simulink model "control_attempt_dofmodel"  (R2020b)
settings: Solver=VariableStepAuto  StartTime=0.0  StopTime=120  FixedStep=0.0001
values from neighbouring files (symbols this model uses):
  g = -9.81    [Variables.m]
undefined symbols (not defined in the file or in its folder): b, ct, Jm, Ke, Kt, L, m, Rm
libraries: pid_lib x2, shared6dof x1
settings Model: Creator=Josh_  LastModifiedBy=maria
settings SolverCC: MaxConsecutiveMinStep=5
settings DataIOCC: SaveFormat=Array  ReturnWorkspaceOutputs=off

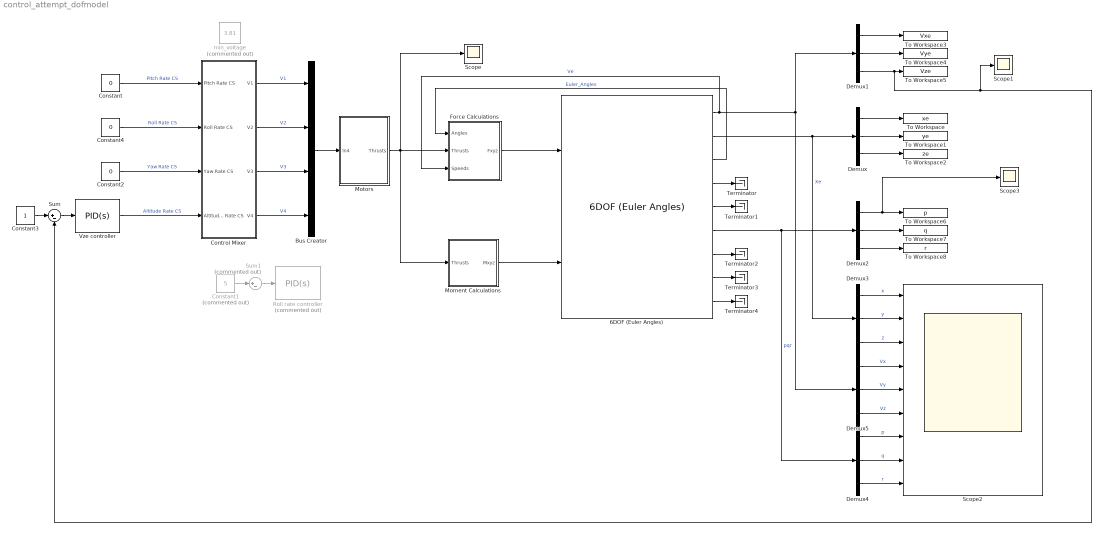
== system control_attempt_dofmodel ==
  6DOF (Euler Angles) : shared6dof/6DOF (Euler Angles)  units=Metric (MKS)  mtype=Fixed  rep=Euler Angles  xme_0=[0 0 0]  Vm_0=[0 0 0]  eul_0=[0 0 0]  pm_0=[0 0 0]  mass_0=m  mass_e=0.5  mass_f=2.0  inertia=eye(3)  inertia_e=eye(3)  inertia_f=2*eye(3)  k_quat=1.0  vre_flag=on  abi_flag=on  aMode=0  xme_statename=''  Vm_statename=''  eul_statename=''  quat_statename=''  pm_statename=''  mass_statename=''
      settings: SourceProductBaseCode=AE,PW,MT,UV,VE,VP
  Bus Creator : BusCreator  Inputs=4
  Constant : Constant  Value=0
  Constant1 : Constant  Commented=on  Value=5
  Constant2 : Constant  Value=0
  Constant3 : Constant
  Constant4 : Constant  Value=0
  Control Mixer : Subsystem
  Demux{,1..5} (6 alike) : Demux  Outputs=3
  Force Calculations : Subsystem
  Moment Calculations : Subsystem
  Motors : Subsystem
  Roll rate controller : pid_lib/PID Controller  Commented=on  Controller=PID  Form=Parallel  TimeDomain=Continuous-time  UseExternalTs=off  SampleTime=-1  IntegratorMethod=Forward Euler  FilterMethod=Forward Euler  ControllerParametersSource=internal  P=249903802210.165  I=8046092299.48993  D=1724573422053.39  UseFilter=on  N=630.713138898879  TunerSelectOption=Transfer Function Based (PID Tuner App)  InitialConditionSource=internal  InitialConditionForIntegrator=0  InitialConditionForFilter=0  DifferentiatorICPrevScaledInput=0  ExternalReset=none  TrackingMode=off  Kt=1  LimitOutput=off  SatLimitsSource=internal  UpperSaturationLimit=inf  LowerSaturationLimit=-inf  LinearizeAsGain=on  AntiWindupMode=none  Kb=1  POutMin=[]  POutMax=[]  IOutMin=[]  IOutMax=[]  DOutMin=[]  DOutMax=[]  NOutMin=[]  NOutMax=[]  SumOutMin=[]  SumOutMax=[]  SaturationOutMin=[]  SaturationOutMax=[]  PParamMin=[]  PParamMax=[]  IParamMin=[]  IParamMax=[]  DParamMin=[]  DParamMax=[]  NParamMin=[]  NParamMax=[]  KbParamMin=[]  KbParamMax=[]  KtParamMin=[]  KtParamMax=[]  KbOutMin=[]  KbOutMax=[]  KtOutMin=[]  KtOutMax=[]  IntegratorOutMin=[]  IntegratorOutMax=[]  FilterOutMin=[]  FilterOutMax=[]  SumI1OutMin=[]  SumI1OutMax=[]  SumI2OutMin=[]  SumI2OutMax=[]  SumI3OutMin=[]  SumI3OutMax=[]  SumI4OutMin=[]  SumI4OutMax=[]  SumDOutMin=[]  SumDOutMax=[]  DifferentiatorOutMin=[]  DifferentiatorOutMax=[]  FilterDiffOutCoefMin=[]  FilterDiffOutCoefMax=[]  ReciprocalOutMin=[]  ReciprocalOutMax=[]  SumDenOutMin=[]  SumDenOutMax=[]  SumNumOutMin=[]  SumNumOutMax=[]  DivideOutMin=[]  DivideOutMax=[]  UdiffTsProdOutMin=[]  UdiffTsProdOutMax=[]  NTsProdOutMin=[]  NTsProdOutMax=[]  UintegralTsProdOutMin=[]  UintegralTsProdOutMax=[]  UngainTsProdOutMin=[]  UngainTsProdOutMax=[]  IntegratorContinuousStateAttributes=''  IntegratorStateMustResolveToSignalObject=off  IntegratorRTWStateStorageClass=Auto  FilterContinuousStateAttributes=''  FilterStateMustResolveToSignalObject=off  FilterRTWStateStorageClass=Auto  ParallelPVariant=InternalParameters  IdealPVariant=Disabled  IVariant=InternalParameters  DVariant=InternalParameters  IntegratorVariant=Continuous  SatVariant=Disabled  AWVariant=Passthrough  PCopyVariant=Disabled  TRVariant=Disabled  FdbkBlocksVariant=Forward  IdealPFdbkVariant=Disabled  SatFdbkVariant=Disabled  DerivativeFilterVariant=ContFilter  NVariant=InternalParameters  NCopyVariant=Disabled  FilterICVariant=InternalICsFilter  IntegratorICVariant=InternalICs  ExternalResetVariant=Disabled  TRSumVariant=Passthrough  SumFdbkVariant=Disabled  SumVariant=Sum_PID  TsampFilterVariant=InternalTs  TsampNgainVariant=Passthrough  TsampIntegralVariant=Passthrough  ExternalSaturationOutDataTypeStr=Inherit: Same as second input
  Scope : Scope
  Scope1 : Scope
  Scope2 : Scope  NumInputPorts=9
  Scope3 : Scope
  Sum : Sum  Inputs=|+-
  Sum1 : Sum  Commented=on  Inputs=|+-
  Terminator{,1..4} (5 alike) : Terminator
  To Workspace : ToWorkspace  VariableName=xe  SampleTime=-1
  To Workspace1 : ToWorkspace  VariableName=ye  SampleTime=-1
  To Workspace2 : ToWorkspace  VariableName=ze  SampleTime=-1
  To Workspace3 : ToWorkspace  VariableName=Vxe  SampleTime=-1
  To Workspace4 : ToWorkspace  VariableName=Vye  SampleTime=-1
  To Workspace5 : ToWorkspace  VariableName=Vze  SampleTime=-1
  To Workspace6 : ToWorkspace  VariableName=p  SampleTime=-1
  To Workspace7 : ToWorkspace  VariableName=q  SampleTime=-1
  To Workspace8 : ToWorkspace  VariableName=r  SampleTime=-1
  Vze controller : pid_lib/PID Controller  Controller=PID  Form=Parallel  TimeDomain=Continuous-time  UseExternalTs=off  SampleTime=-1  IntegratorMethod=Forward Euler  FilterMethod=Forward Euler  ControllerParametersSource=internal  P=0.555  I=0.018  D=3.728  UseFilter=on  N=647.736587390862  TunerSelectOption=Transfer Function Based (PID Tuner App)  InitialConditionSource=internal  InitialConditionForIntegrator=0  InitialConditionForFilter=0  DifferentiatorICPrevScaledInput=0  ExternalReset=none  TrackingMode=off  Kt=1  LimitOutput=off  SatLimitsSource=internal  UpperSaturationLimit=inf  LowerSaturationLimit=-inf  LinearizeAsGain=on  AntiWindupMode=none  Kb=1  POutMin=[]  POutMax=[]  IOutMin=[]  IOutMax=[]  DOutMin=[]  DOutMax=[]  NOutMin=[]  NOutMax=[]  SumOutMin=[]  SumOutMax=[]  SaturationOutMin=[]  SaturationOutMax=[]  PParamMin=[]  PParamMax=[]  IParamMin=[]  IParamMax=[]  DParamMin=[]  DParamMax=[]  NParamMin=[]  NParamMax=[]  KbParamMin=[]  KbParamMax=[]  KtParamMin=[]  KtParamMax=[]  KbOutMin=[]  KbOutMax=[]  KtOutMin=[]  KtOutMax=[]  IntegratorOutMin=[]  IntegratorOutMax=[]  FilterOutMin=[]  FilterOutMax=[]  SumI1OutMin=[]  SumI1OutMax=[]  SumI2OutMin=[]  SumI2OutMax=[]  SumI3OutMin=[]  SumI3OutMax=[]  SumI4OutMin=[]  SumI4OutMax=[]  SumDOutMin=[]  SumDOutMax=[]  DifferentiatorOutMin=[]  DifferentiatorOutMax=[]  FilterDiffOutCoefMin=[]  FilterDiffOutCoefMax=[]  ReciprocalOutMin=[]  ReciprocalOutMax=[]  SumDenOutMin=[]  SumDenOutMax=[]  SumNumOutMin=[]  SumNumOutMax=[]  DivideOutMin=[]  DivideOutMax=[]  UdiffTsProdOutMin=[]  UdiffTsProdOutMax=[]  NTsProdOutMin=[]  NTsProdOutMax=[]  UintegralTsProdOutMin=[]  UintegralTsProdOutMax=[]  UngainTsProdOutMin=[]  UngainTsProdOutMax=[]  IntegratorContinuousStateAttributes=''  IntegratorStateMustResolveToSignalObject=off  IntegratorRTWStateStorageClass=Auto  FilterContinuousStateAttributes=''  FilterStateMustResolveToSignalObject=off  FilterRTWStateStorageClass=Auto  ParallelPVariant=InternalParameters  IdealPVariant=Disabled  IVariant=InternalParameters  DVariant=InternalParameters  IntegratorVariant=Continuous  SatVariant=Disabled  AWVariant=Passthrough  PCopyVariant=Disabled  TRVariant=Disabled  FdbkBlocksVariant=Forward  IdealPFdbkVariant=Disabled  SatFdbkVariant=Disabled  DerivativeFilterVariant=ContFilter  NVariant=InternalParameters  NCopyVariant=Disabled  FilterICVariant=InternalICsFilter  IntegratorICVariant=InternalICs  ExternalResetVariant=Disabled  TRSumVariant=Passthrough  SumFdbkVariant=Disabled  SumVariant=Sum_PID  TsampFilterVariant=InternalTs  TsampNgainVariant=Passthrough  TsampIntegralVariant=Passthrough  ExternalSaturationOutDataTypeStr=Inherit: Same as second input
  min_voltage : Constant  Commented=on  Value=3.81
  wires:
  Demux4/1 -> Scope2/7  "p"
  Demux3/3 -> Scope2/3  "z"
  Demux4/2 -> Scope2/8  "q"
  Demux4/3 -> Scope2/9  "r"
  Demux5/2 -> Scope2/5  "Vy"
  Demux2/1 -> Scope3/1, To Workspace6/1
  Demux3/2 -> Scope2/2  "y"
  Constant/1 -> Control Mixer/1(Pitch Rate CS)  "Pitch Rate CS"
  Vze controller/1 -> Control Mixer/4(Altitude Rate CS)  "Altitude Rate CS"
  Demux3/1 -> Scope2/1  "x"
  6DOF (Euler Angles)/6 -> Demux4/1, Demux2/1  "pqr"
  Demux5/1 -> Scope2/4  "Vx"
  Demux2/3 -> To Workspace8/1
  Demux2/2 -> To Workspace7/1
  Control Mixer/4(V4) -> Bus Creator/4  "V4"
  Demux5/3 -> Scope2/6  "Vz"
  Control Mixer/3(V3) -> Bus Creator/3  "V3"
  Demux/1 -> To Workspace/1
  Constant2/1 -> Control Mixer/3(Yaw Rate CS)  "Yaw Rate CS"
  Demux1/2 -> To Workspace4/1
  Demux1/1 -> To Workspace3/1
  Motors/1(Thrusts) -> Moment Calculations/1(Thrusts), Force Calculations/2(Thrusts), Scope/1
  Control Mixer/1(V1) -> Bus Creator/1  "V1"
  Demux1/3 -> Scope1/1, Sum/2, To Workspace5/1
  Control Mixer/2(V2) -> Bus Creator/2  "V2"
  Bus Creator/1 -> Motors/1(In4)
  Demux/3 -> To Workspace2/1
  Force Calculations/1(Fxyz) -> 6DOF (Euler Angles)/1
  Demux/2 -> To Workspace1/1
  6DOF (Euler Angles)/2 -> Demux3/1, Demux/1  "Xe"
  Moment Calculations/1(Mxyz) -> 6DOF (Euler Angles)/2
  6DOF (Euler Angles)/3 -> Force Calculations/1(Angles)  "Euler_Angles"
  6DOF (Euler Angles)/1 -> Force Calculations/3(Speeds), Demux5/1, Demux1/1  "Ve"
  Constant3/1 -> Sum/1
  Sum/1 -> Vze controller/1
  6DOF (Euler Angles)/4 -> Terminator/1
  6DOF (Euler Angles)/5 -> Terminator1/1
  6DOF (Euler Angles)/7 -> Terminator2/1
  6DOF (Euler Angles)/8 -> Terminator3/1
  6DOF (Euler Angles)/9 -> Terminator4/1
  Sum1/1 -> Roll rate controller/1
  Constant1/1 -> Sum1/1
  Constant4/1 -> Control Mixer/2(Roll Rate CS)  "Roll Rate CS"

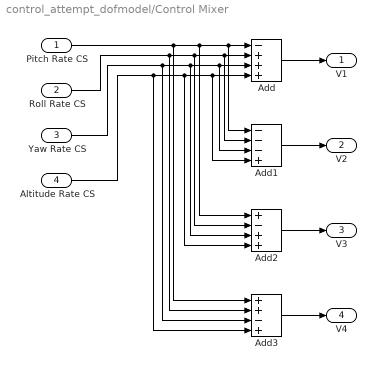
== system control_attempt_dofmodel/Control Mixer ==
  Pitch Rate CS : Inport
  Roll Rate CS : Inport  Port=2
  Yaw Rate CS : Inport  Port=3
  Altitude Rate CS : Inport  Port=4
  Add : Sum  Inputs=-+++
  Add1 : Sum  Inputs=---+
  Add2 : Sum  Inputs=+-++
  Add3 : Sum  Inputs=++-+
  V1 : Outport
  V2 : Outport  Port=2
  V3 : Outport  Port=3
  V4 : Outport  Port=4
  wires:
  Pitch Rate CS/1 -> Add1/1, Add/1, Add2/1, Add3/1
  Roll Rate CS/1 -> Add1/2, Add/2, Add2/2, Add3/2
  Yaw Rate CS/1 -> Add3/3, Add1/3, Add/3, Add2/3
  Altitude Rate CS/1 -> Add2/4, Add1/4, Add/4, Add3/4
  Add/1 -> V1/1
  Add1/1 -> V2/1
  Add2/1 -> V3/1
  Add3/1 -> V4/1

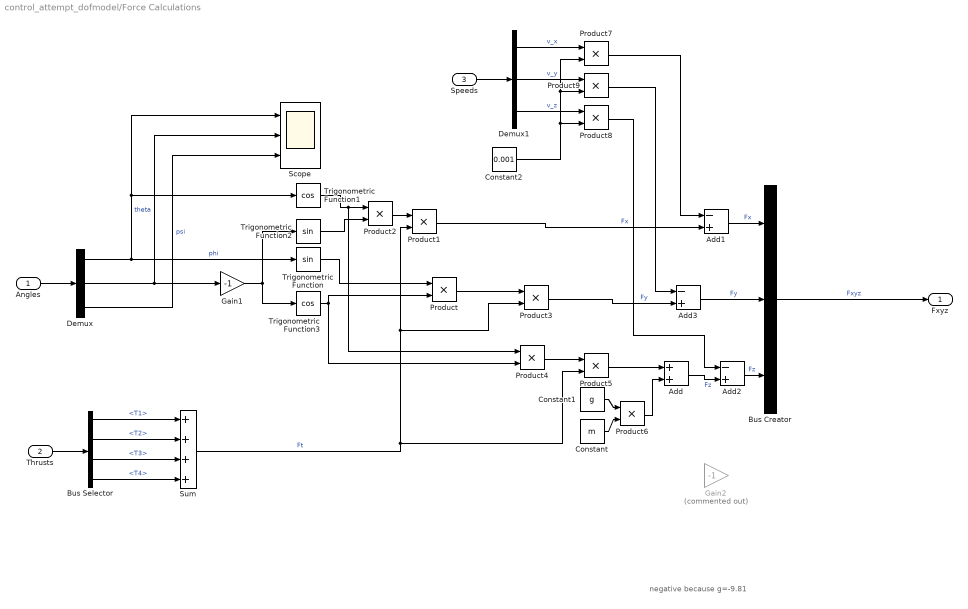
== system control_attempt_dofmodel/Force Calculations ==
  note: negative because g=-9.81
  Angles : Inport
  Thrusts : Inport  Port=2
  Speeds : Inport  Port=3
  Add : Sum
  Add1 : Sum  Inputs=-+
  Add2 : Sum  Inputs=-+
  Add3 : Sum  Inputs=-+
  Bus Creator : BusCreator  Inputs=3
  Bus Selector : BusSelector  OutputSignals=T1,T2,T3,T4
  Constant : Constant  Value=m
  Constant1 : Constant  Value=g
  Constant2 : Constant  Value=0.001
  Demux : Demux  Outputs=3
  Demux1 : Demux  Outputs=3
  Gain1 : Gain  Gain=-1
  Gain2 : Gain  Commented=on  Gain=-1
  Product{,1..9} (10 alike) : Product
  Scope : Scope  NumInputPorts=3
  Sum : Sum  Inputs=++++
  Trigonometric Function : Trigonometry
  Trigonometric Function1 : Trigonometry  Operator=cos
  Trigonometric Function2 : Trigonometry
  Trigonometric Function3 : Trigonometry  Operator=cos
  Fxyz : Outport
  wires:
  Constant/1 -> Product6/2
  Constant1/1 -> Product6/1
  Product5/1 -> Add/1
  Product4/1 -> Product5/1
  Product/1 -> Product3/1
  Demux/2 -> Gain1/1, Scope/2  "theta"
  Demux/1 -> Trigonometric Function/1, Trigonometric Function1/1, Scope/1  "phi"
  Angles/1 -> Demux/1
  Demux/3 -> Scope/3  "psi"
  Gain1/1 -> Trigonometric Function2/1, Trigonometric Function3/1
  Trigonometric Function1/1 -> Product4/1, Product2/1
  Trigonometric Function2/1 -> Product2/2
  Product2/1 -> Product1/1
  Sum/1 -> Product5/2, Product1/2, Product3/2  "Ft"
  Trigonometric Function/1 -> Product/1
  Trigonometric Function3/1 -> Product4/2, Product/2
  Thrusts/1 -> Bus Selector/1
  Bus Selector/1 -> Sum/1  "<T1>"
  Bus Selector/2 -> Sum/2  "<T2>"
  Bus Selector/3 -> Sum/3  "<T3>"
  Bus Selector/4 -> Sum/4  "<T4>"
  Bus Creator/1 -> Fxyz/1  "Fxyz"
  Product6/1 -> Add/2
  Speeds/1 -> Demux1/1
  Demux1/1 -> Product7/1  "v_x"
  Demux1/2 -> Product9/1  "v_y"
  Demux1/3 -> Product8/1  "v_z"
  Constant2/1 -> Product8/2, Product9/2, Product7/2
  Product1/1 -> Add1/2  "Fx"
  Add1/1 -> Bus Creator/1  "Fx"
  Add/1 -> Add2/2  "Fz"
  Add2/1 -> Bus Creator/3  "Fz"
  Add3/1 -> Bus Creator/2  "Fy"
  Product3/1 -> Add3/2  "Fy"
  Product8/1 -> Add2/1
  Product9/1 -> Add3/1
  Product7/1 -> Add1/1

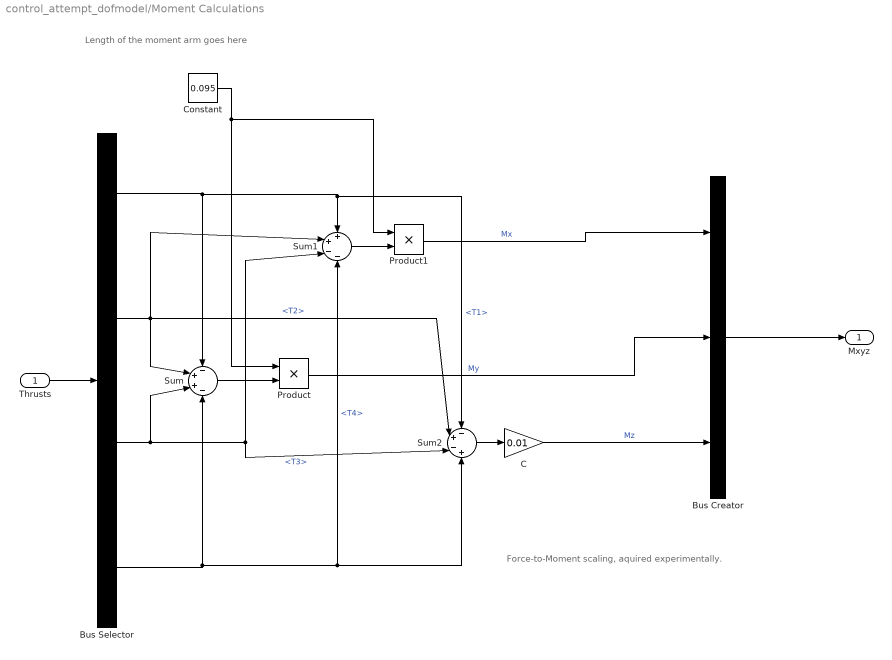
== system control_attempt_dofmodel/Moment Calculations ==
  note: Length of the moment arm goes here
  note: Force-to-Moment scaling, aquired experimentally.
  Thrusts : Inport
  Bus Creator : BusCreator  Inputs=3
  Bus Selector : BusSelector  OutputSignals=T1,T2,T3,T4
  C : Gain  Gain=0.01
  Constant : Constant  Value=0.095
  Product : Product
  Product1 : Product
  Sum : Sum  Inputs=-++-
  Sum1 : Sum  Inputs=++--
  Sum2 : Sum  Inputs=-+-+
  Mxyz : Outport
  wires:
  Bus Creator/1 -> Mxyz/1
  Bus Selector/1 -> Sum2/1, Sum1/1, Sum/1  "<T1>"
  Bus Selector/4 -> Sum2/4, Sum1/4, Sum/4  "<T4>"
  Thrusts/1 -> Bus Selector/1
  Bus Selector/2 -> Sum2/2, Sum/2, Sum1/2  "<T2>"
  Bus Selector/3 -> Sum1/3, Sum2/3, Sum/3  "<T3>"
  Sum2/1 -> C/1
  C/1 -> Bus Creator/3  "Mz"
  Sum/1 -> Product/2
  Constant/1 -> Product1/1, Product/1
  Sum1/1 -> Product1/2
  Product1/1 -> Bus Creator/1  "Mx"
  Product/1 -> Bus Creator/2  "My"

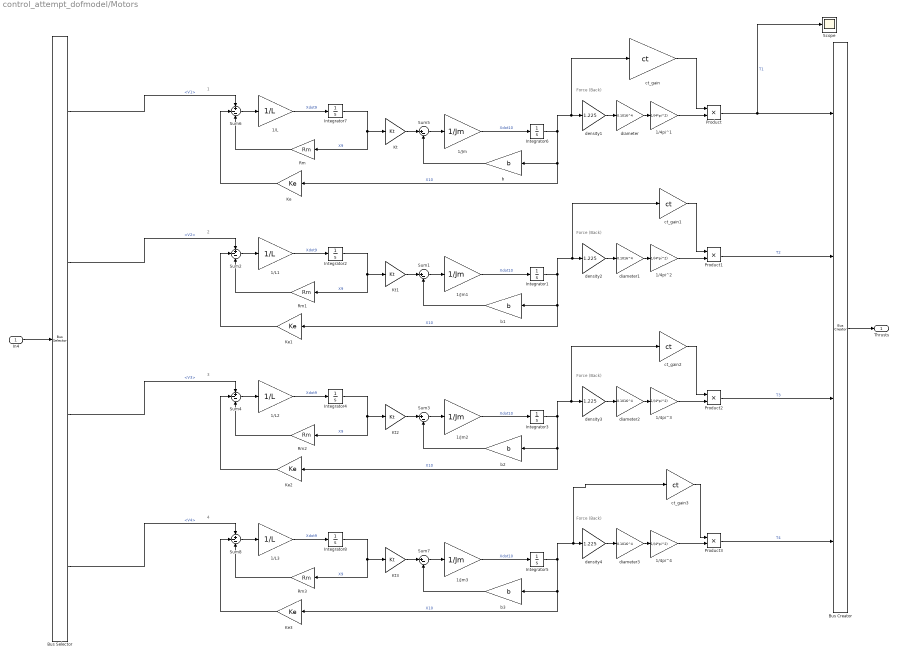
== system control_attempt_dofmodel/Motors ==
  note: Force (Back)
  note: 1
  note: 2
  note: Force (Back)
  note: 3
  note: Force (Back)
  note: 4
  note: Force (Back)
  In4 : Inport
  1/4pi^{1..4} (4 alike) : Gain  Gain=1/(4*pi^2)
  1/Jm{,1..3} (4 alike) : Gain  Gain=1/Jm
  1/L{,1..3} (4 alike) : Gain  Gain=1/L
  Bus Creator : BusCreator  Inputs=4
  Bus Selector : BusSelector  OutputSignals=V1,V2,V3,V4
  Integrator{1..8} (8 alike) : Integrator
  Ke{,1..3} (4 alike) : Gain  Gain=Ke
  Kt{,1..3} (4 alike) : Gain  Gain=Kt
  Product{,1..3} (4 alike) : Product
  Rm{,1..3} (4 alike) : Gain  Gain=Rm
  Scope : Scope
  Sum{1,3,5,7} (4 alike) : Sum  Inputs=|+-
  Sum{2,4,6,8} (4 alike) : Sum  Inputs=+--
  b{,1..3} (4 alike) : Gain  Gain=b
  ct_gain{,1..3} (4 alike) : Gain  Gain=ct
  density{1..4} (4 alike) : Gain  Gain=1.225
  diameter{,1..3} (4 alike) : Gain  Gain=0.1016^4
  Thrusts : Outport
  wires:
  In4/1 -> Bus Selector/1
  Sum5/1 -> 1/Jm/1
  Rm/1 -> Sum6/3
  1/Jm/1 -> Integrator6/1  "Xdot10"
  1/L/1 -> Integrator7/1  "Xdot9"
  diameter/1 -> 1/4pi^1/1
  Integrator6/1 -> density1/1, ct_gain/1, b/1, Ke/1  "X10"
  1/4pi^1/1 -> Product/2
  Integrator7/1 -> Rm/1, Kt/1  "X9"
  Kt/1 -> Sum5/1
  density1/1 -> diameter/1
  b/1 -> Sum5/2
  Sum6/1 -> 1/L/1
  Ke/1 -> Sum6/2
  Bus Creator/1 -> Thrusts/1
  b1/1 -> Sum1/2
  Ke1/1 -> Sum2/2
  Integrator2/1 -> Rm1/1, Kt1/1  "X9"
  density2/1 -> diameter1/1
  Sum2/1 -> 1/L1/1
  1/4pi^2/1 -> Product1/2
  1/Jm1/1 -> Integrator1/1  "Xdot10"
  diameter1/1 -> 1/4pi^2/1
  Kt1/1 -> Sum1/1
  1/L1/1 -> Integrator2/1  "Xdot9"
  Rm1/1 -> Sum2/3
  Sum1/1 -> 1/Jm1/1
  b2/1 -> Sum3/2
  Ke2/1 -> Sum4/2
  Integrator4/1 -> Rm2/1, Kt2/1  "X9"
  density3/1 -> diameter2/1
  Sum4/1 -> 1/L2/1
  1/4pi^3/1 -> Product2/2
  1/Jm2/1 -> Integrator3/1  "Xdot10"
  diameter2/1 -> 1/4pi^3/1
  Kt2/1 -> Sum3/1
  1/L2/1 -> Integrator4/1  "Xdot9"
  Rm2/1 -> Sum4/3
  Sum3/1 -> 1/Jm2/1
  b3/1 -> Sum7/2
  Ke3/1 -> Sum8/2
  Integrator8/1 -> Rm3/1, Kt3/1  "X9"
  density4/1 -> diameter3/1
  Sum8/1 -> 1/L3/1
  1/4pi^4/1 -> Product3/2
  1/Jm3/1 -> Integrator5/1  "Xdot10"
  diameter3/1 -> 1/4pi^4/1
  Kt3/1 -> Sum7/1
  1/L3/1 -> Integrator8/1  "Xdot9"
  Rm3/1 -> Sum8/3
  Sum7/1 -> 1/Jm3/1
  ct_gain/1 -> Product/1
  Product/1 -> Scope/1, Bus Creator/1  "T1"
  Product1/1 -> Bus Creator/2  "T2"
  Product2/1 -> Bus Creator/3  "T3"
  Product3/1 -> Bus Creator/4  "T4"
  Integrator1/1 -> ct_gain1/1, density2/1, b1/1, Ke1/1  "X10"
  ct_gain1/1 -> Product1/1
  Integrator3/1 -> ct_gain2/1, density3/1, b2/1, Ke2/1  "X10"
  ct_gain2/1 -> Product2/1
  Integrator5/1 -> ct_gain3/1, density4/1, b3/1, Ke3/1  "X10"
  ct_gain3/1 -> Product3/1
  Bus Selector/1 -> Sum6/1  "<V1>"
  Bus Selector/2 -> Sum2/1  "<V2>"
  Bus Selector/3 -> Sum4/1  "<V3>"
  Bus Selector/4 -> Sum8/1  "<V4>"
